simulink model "modelo_f_HIL"  (R2024b)
settings: Solver=ode15s  StartTime=0.0  StopTime=inf  FixedStep=T_s  RelTol=1e-3
InitFcn:
  | clc
  | clear
  | close all
  | clear all
  | clear mex
  | parametros
  | gain_CL
  | calculo_observador_carro
  | calculo_observador_izaje
values from neighbouring files (symbols this model uses):
  b_cx = 1e6    (= 1000000)    [parametros.m]
  b_cy = 1e7    (= 10000000)    [parametros.m]
  b_hb = 1e8    (= 100000000)    [parametros.m]
  b_hd = 8    [parametros.m]
  b_hm = 18    [parametros.m]
  b_t = 90    [parametros.m]
  b_tb = 5e6    (= 5000000)    [parametros.m]
  b_td = 1.8    [parametros.m]
  b_tm = 6    [parametros.m]
  b_tw = 3e3    (= 3000)    [parametros.m]
  b_wu = 150    [parametros.m]
  container_pillars = container_pillars(randperm(19))    [parametros.m]
  escenario = 1    [parametros.m]
  g = 9.80665    [parametros.m]
  H_c = 2.59    [parametros.m]
  H_truck = 1    [parametros.m]
  i_h = 22    [parametros.m]
  i_t = 30    [parametros.m]
  J_hd_hEb = 3800    [parametros.m]
  J_hm_hb = 30    [parametros.m]
  J_td = 1200    [parametros.m]
  J_tm_tb = 7    [parametros.m]
  K_cy = 1.8e9    (= 1800000000)    [parametros.m]
  K_tw = 4.8e5    (= 480000)    [parametros.m]
  k_wu = 2.36e8    (= 236000000)    [parametros.m]
  l_h0 = (Y_t0-y_l0)    (= 15)    [parametros.m]
  l_h_max = Y_t0-y_h_min    (= 65)    [parametros.m]
  l_h_maxE = l_h_max+0.5    (= 65.5)    [parametros.m]
  l_h_min = Y_t0-y_h_max    (= 5)    [parametros.m]
  l_h_minE = l_h_min-0.5    (= 4.5)    [parametros.m]
  M_cmax = 50000    [parametros.m]
  M_cmin = 2000    [parametros.m]
  M_s = 15000    [parametros.m]
  M_t = 30000    [parametros.m]
  r_hd = 0.75    [parametros.m]
  r_td = 0.50    (= 0.5)    [parametros.m]
  T_hbMax = 5e4    (= 50000)    [parametros.m]
  T_hEbMax = 1.1e6    (= 1100000)    [parametros.m]
  T_hmMax = 2e4    (= 20000)    [parametros.m]
  T_s = 0.001    [parametros.m]
  T_s0 = 0.001    [parametros.m]
  T_s1 = 0.020    (= 0.02)    [parametros.m]
  T_s2 = 0.020    (= 0.02)    [parametros.m]
  T_tbMax = 5e3    (= 5000)    [parametros.m]
  T_tmMax = 4e3    (= 4000)    [parametros.m]
  tau_tm = 1e-3    (= 0.001)    [parametros.m]
  theta_hm0 = -l_h0*i_h*2/r_hd    (= -880)    [parametros.m]
  theta_tm0 = (x_t0)*i_t/r_td    (= -1500)    [parametros.m]
  trucks0 = [0, 0, 0, 0, 0]    [parametros.m]
  v_h_max_load = 1.5    [parametros.m]
  v_h_max_noload = 3    [parametros.m]
  v_lx0 = 0    [parametros.m]
  v_ly0 = 0    [parametros.m]
  v_t0 = 0    [parametros.m]
  v_t_max = 4    [parametros.m]
  W_c = ctrb(A, B_c(:,1))    [CyO_carro.m]    (also in CyO_izaje.m; parametros.m = 2.44)
  w_hm0 = 0    [parametros.m]
  w_hm_rated = v_h_max_load*2*i_h/r_hd    (= 88)    [parametros.m]
  w_tm0 = (v_t0)*i_t/r_td    (= 0)    [parametros.m]
  x_c0_left = -35    [parametros.m]
  x_c0_right = 55    [parametros.m]
  x_containers_left_lim = 1.5    [parametros.m]
  x_containers_right_lim = 48.5    [parametros.m]
  x_l0 = x_t0    (= -25)    [parametros.m]
  x_lidar_offset = 3.0    (= 3)    [parametros.m]
  x_t0 = -25    [parametros.m]
  x_t_max = 50    [parametros.m]
  x_t_maxE = x_t_max+0.5    (= 50.5)    [parametros.m]
  x_t_min = -30    [parametros.m]
  x_t_minE = x_t_min-0.5    (= -30.5)    [parametros.m]
  y_h_min = -20    [parametros.m]
  y_l0 = 30    [parametros.m]
  Y_sb = 5.0    (= 5)    [parametros.m]
  Y_t0 = 45    [parametros.m]
libraries: opcualib x2, dspnetwork x2, dspsigops x1, simulink x1
(part 1 of 3)
settings Model: Creator=Usuario  LastModifiedBy=Usuario
settings RTWCC: GPUComputeCapability=3.5

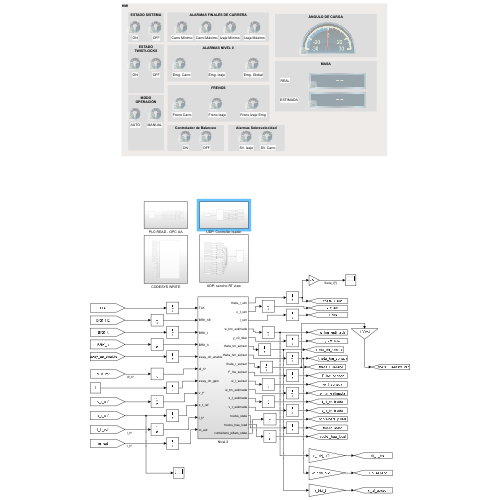
[thumbnail: Simulink's stored preview of the top-level diagram]
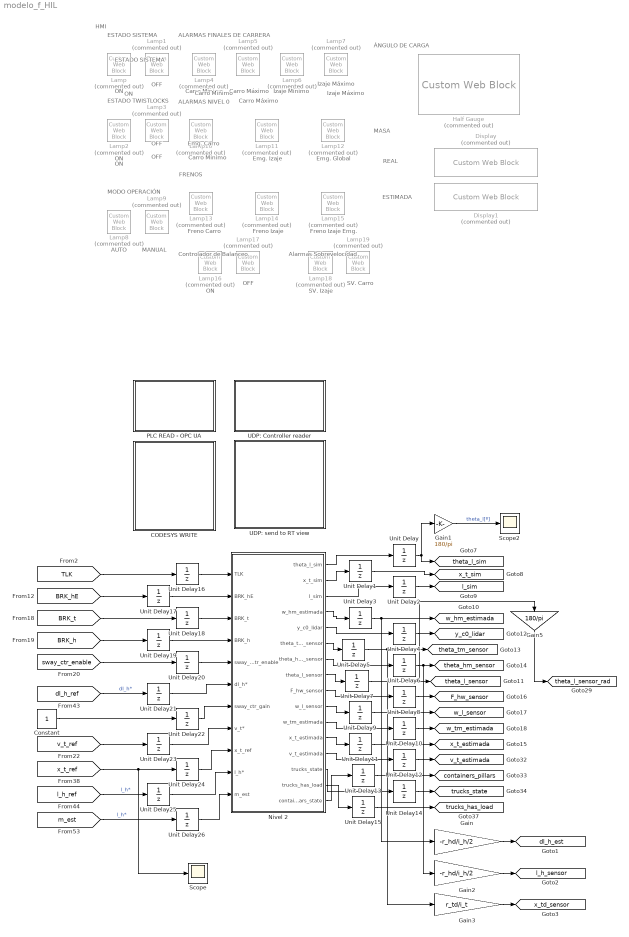
== system modelo_f_HIL ==
  note: ESTIMADA
  note: REAL
  note: OFF
  note: ON
  note: ESTADO SISTEMA
  note: HMI
  note: ON
  note: ESTADO SISTEMA
  note: ESTADO TWISTLOCKS
  note: OFF
  note: ON
  note: ON
  note: OFF
  note: Carro Mínimo
  note: ALARMAS FINALES DE CARRERA
  note: Carro Máximo
  note: Izaje Mínimo
  note: Izaje Máximo
  note: MANUAL
  note: AUTO
  note: MODO
      | OPERACIÓN
  note: Emg. Izaje
  note: ALARMAS NIVEL 0
  note: Carro Mínimo
  note: Izaje Máximo
  note: Carro Máximo
  note: Carro Mínimo
  note: Emg. Carro
  note: Emg. Global
  note: Freno Izaje Emg.
  note: Freno Carro
  note: FRENOS
  note: Freno Izaje
  note: OFF
  note: ON
  note: Controlador de Balanceo
  note: ÁNGULO DE CARGA
  note: MASA
  note: Alarmas Sobrevelocidad
  note: SV. Izaje
  note: SV. Carro
  CODESYS WRITE : Subsystem
  Constant : Constant
  Display : CustomWebBlock  Commented=on  LabelPosition=Hide  ShowInitialText=on  Configuration="{\"components\":[{\"name\":\"DisplayComponent\",\"settings\":{\"bold\":false,\"font\":\"DSEG7 Classic\",\"fontColor\":[255,255,200],\"fontSize\":\"14\",\"format\":\"short\",\"formatString\":\"%d\",\"italic\":false,\"position\":[0,0,1,1],\"underline\":false}},{\"name\":\"BackgroundImageComponent\",\"settings\":{\"image\":{\"size\":[300,80],\"src\":\"data:image\\/svg+xml;base64,PHN2ZyBpZD0iZnJhbWUiIHhtbG5zPSJodHRwOi8vd3d3LnczLm9yZy8yMDAwL3N2ZyIgeG1sbnM6eGxpbms9Imh0dHA6Ly93d3cudzMub3JnLzE5OTkveGxpbmsiIHZpZXdCb3g9IjAgMCAzODAgMTAxIj48ZGVmcz48c3R5bGU+LmNscy0xe2ZpbGw6IzAwMmI0Mjt9LmNscy0ye2ZpbGw6IzQyNzA4Mjt9LmNscy0ze2ZpbGw6dXJsKCNyYWRpYWwtZ3JhZGllbnQpO308L3N0eWxlPjxyYWRpYWxHcmFkaWVudCBpZD0icmFkaWFsLWdyYWRpZW50IiBjeD0iMTkwIiBjeT0iNTAuNSIgcj0iMjY5LjIxIiBncmFkaWVudFVuaXRzPSJ1c2VyU3BhY2VPblVzZSI+PHN0b3Agb2Zmc2V0PSIwLjAxIiBzdG9wLWNvbG9yPSIjM2U0ZjU4Ii8+PHN0b3Agb2Zmc2V0PSIwLjA2IiBzdG9wLWNvbG9yPSIjNDQ1NzYxIi8+PHN0b3Agb2Zmc2V0PSIwLjE1IiBzdG9wLWNvbG9yPSIjNTU2YTc2Ii8+PHN0b3Agb2Zmc2V0PSIwLjI1IiBzdG9wLWNvbG9yPSIjNmQ4ODk1Ii8+PHN0b3Agb2Zmc2V0PSIwLjM4IiBzdG9wLWNvbG9yPSIjOGZiMmMzIi8+PHN0b3Agb2Zmc2V0PSIwLjUyIiBzdG9wLWNvbG9yPSIjYjZlNGZhIi8+PHN0b3Agb2Zmc2V0PSIxIiBzdG9wLWNvbG9yPSIjMTU0NjU3Ii8+PC9yYWRpYWxHcmFkaWVudD48L2RlZnM+PGcgaWQ9IkxheWVyXzIiIGRhdGEtbmFtZT0iTGF5ZXIgMiI+PGcgaWQ9IkxheWVyXzEtMiIgZGF0YS1uYW1lPSJMYXllciAxLTIiPjxyZWN0IGlkPSJyZWN0MTAzNiIgY2xhc3M9ImNscy0xIiB4PSIxMSIgeT0iMTEiIHdpZHRoPSIzNTgiIGhlaWdodD0iNzkiLz48cGF0aCBpZD0icGF0aDEwMzgiIGNsYXNzPSJjbHMtMiIgZD0iTTgsOFY5M0gzNzJWOFpNMzY5LDkwSDExVjExSDM2OVoiLz48cGF0aCBpZD0icGF0aDEwNDAiIGNsYXNzPSJjbHMtMyIgZD0iTTAsMFYxMDFIMzgwVjBaTTM3Miw5M0g4VjhIMzcyWiIvPjwvZz48L2c+PC9zdmc+\",\"srcOrientation\":\"Right\"},\"position\":[0,0,1,1],\"scaleMode\":\"0\"}},{\"name\":\"ForegroundImageComponent\",\"settings\":{\"angle\":0,\"image\":{\"size\":[0,0],\"src\":\"default\"},\"isForeground\":1,\"position\":[0,0,1,1],\"scaleMode\":\"0\"}}],\"settings\":{\"BindingType\":\"signal\",\"aspectRatio\":1.032258064516129,\"backgroundColor\":[0,0,0,\"1\"],\"backgroundOffset\":0.14,\"backgroundOpacity\":1,\"fixedAspectRatio\":\"on\",\"showBackgroundColor\":false,\"value\":0,\"version\":\"R2023b\"},\"type\":\"Display\"}"
  Display1 : CustomWebBlock  Commented=on  LabelPosition=Hide  ShowInitialText=on  Configuration="{\"components\":[{\"name\":\"DisplayComponent\",\"settings\":{\"bold\":false,\"font\":\"DSEG7 Classic\",\"fontColor\":[255,255,200],\"fontSize\":\"14\",\"format\":\"short\",\"formatString\":\"%d\",\"italic\":false,\"position\":[0,0,1,1],\"underline\":false}},{\"name\":\"BackgroundImageComponent\",\"settings\":{\"image\":{\"size\":[300,80],\"src\":\"data:image\\/svg+xml;base64,PHN2ZyBpZD0iZnJhbWUiIHhtbG5zPSJodHRwOi8vd3d3LnczLm9yZy8yMDAwL3N2ZyIgeG1sbnM6eGxpbms9Imh0dHA6Ly93d3cudzMub3JnLzE5OTkveGxpbmsiIHZpZXdCb3g9IjAgMCAzODAgMTAxIj48ZGVmcz48c3R5bGU+LmNscy0xe2ZpbGw6IzAwMmI0Mjt9LmNscy0ye2ZpbGw6IzQyNzA4Mjt9LmNscy0ze2ZpbGw6dXJsKCNyYWRpYWwtZ3JhZGllbnQpO308L3N0eWxlPjxyYWRpYWxHcmFkaWVudCBpZD0icmFkaWFsLWdyYWRpZW50IiBjeD0iMTkwIiBjeT0iNTAuNSIgcj0iMjY5LjIxIiBncmFkaWVudFVuaXRzPSJ1c2VyU3BhY2VPblVzZSI+PHN0b3Agb2Zmc2V0PSIwLjAxIiBzdG9wLWNvbG9yPSIjM2U0ZjU4Ii8+PHN0b3Agb2Zmc2V0PSIwLjA2IiBzdG9wLWNvbG9yPSIjNDQ1NzYxIi8+PHN0b3Agb2Zmc2V0PSIwLjE1IiBzdG9wLWNvbG9yPSIjNTU2YTc2Ii8+PHN0b3Agb2Zmc2V0PSIwLjI1IiBzdG9wLWNvbG9yPSIjNmQ4ODk1Ii8+PHN0b3Agb2Zmc2V0PSIwLjM4IiBzdG9wLWNvbG9yPSIjOGZiMmMzIi8+PHN0b3Agb2Zmc2V0PSIwLjUyIiBzdG9wLWNvbG9yPSIjYjZlNGZhIi8+PHN0b3Agb2Zmc2V0PSIxIiBzdG9wLWNvbG9yPSIjMTU0NjU3Ii8+PC9yYWRpYWxHcmFkaWVudD48L2RlZnM+PGcgaWQ9IkxheWVyXzIiIGRhdGEtbmFtZT0iTGF5ZXIgMiI+PGcgaWQ9IkxheWVyXzEtMiIgZGF0YS1uYW1lPSJMYXllciAxLTIiPjxyZWN0IGlkPSJyZWN0MTAzNiIgY2xhc3M9ImNscy0xIiB4PSIxMSIgeT0iMTEiIHdpZHRoPSIzNTgiIGhlaWdodD0iNzkiLz48cGF0aCBpZD0icGF0aDEwMzgiIGNsYXNzPSJjbHMtMiIgZD0iTTgsOFY5M0gzNzJWOFpNMzY5LDkwSDExVjExSDM2OVoiLz48cGF0aCBpZD0icGF0aDEwNDAiIGNsYXNzPSJjbHMtMyIgZD0iTTAsMFYxMDFIMzgwVjBaTTM3Miw5M0g4VjhIMzcyWiIvPjwvZz48L2c+PC9zdmc+\",\"srcOrientation\":\"Right\"},\"position\":[0,0,1,1],\"scaleMode\":\"0\"}},{\"name\":\"ForegroundImageComponent\",\"settings\":{\"angle\":0,\"image\":{\"size\":[0,0],\"src\":\"default\"},\"isForeground\":1,\"position\":[0,0,1,1],\"scaleMode\":\"0\"}}],\"settings\":{\"BindingType\":\"signal\",\"aspectRatio\":1.032258064516129,\"backgroundColor\":[0,0,0,\"1\"],\"backgroundOffset\":0.14,\"backgroundOpacity\":1,\"fixedAspectRatio\":\"on\",\"showBackgroundColor\":false,\"value\":0,\"version\":\"R2023b\"},\"type\":\"Display\"}"
  Gain : Gain  Gain=-r_hd/i_h/2
  Gain1 : Gain  Gain=180/pi
  Gain2 : Gain  Gain=-r_hd/i_h/2
  Gain3 : Gain  Gain=r_td/i_t
  Gain5 : Gain  Gain=180/pi
  Half Gauge : CustomWebBlock  Commented=on  LabelPosition=Hide  ShowInitialText=on  Configuration="{\"components\":[{\"name\":\"CircularScaleComponent\",\"settings\":{\"bounds\":{\"max\":30,\"min\":-30,\"tickInterval\":\"auto\"},\"direction\":\"cw\",\"flipLimits\":0,\"innerRadius\":0.75,\"internalTickHeightScaleFactor\":1,\"labelColor\":[255,255,200],\"labelFont\":{\"font\":\"Arial\",\"fontSize\":12},\"labelRadius\":0.528,\"labelTransparency\":1,\"minorTickHeightScaleFactor\":0.2,\"needleImage\":{\"size\":[200,50],\"src\":\"data:image\\/svg+xml;base64,PD94bWwgdmVyc2lvbj0iMS4wIiBlbmNvZGluZz0idXRmLTgiPz4KPCEtLSBHZW5lcmF0b3I6IEFkb2JlIElsbHVzdHJhdG9yIDI0LjEuMiwgU1ZHIEV4cG9ydCBQbHVnLUluIC4gU1ZHIFZlcnNpb246IDYuMDAgQnVpbGQgMCkgIC0tPgo8c3ZnIHZlcnNpb249IjEuMSIgaWQ9IkxheWVyXzEiIHhtbG5zPSJodHRwOi8vd3d3LnczLm9yZy8yMDAwL3N2ZyIgeG1sbnM6eGxpbms9Imh0dHA6Ly93d3cudzMub3JnLzE5OTkveGxpbmsiIHg9IjBweCIgeT0iMHB4IgoJIHZpZXdCb3g9IjAgMCAyMDAgNTAiIHN0eWxlPSJlbmFibGUtYmFja2dyb3VuZDpuZXcgMCAwIDIwMCA1MDsiIHhtbDpzcGFjZT0icHJlc2VydmUiPgo8c3R5bGUgdHlwZT0idGV4dC9jc3MiPgoJLnN0MHtmaWxsOiNFQzIxMjc7fQo8L3N0eWxlPgo8cGF0aCBjbGFzcz0ic3QwIiBkPSJNMTYyLjgsMTMuN0MxNjksNC40LDE4MS43LDEuOSwxOTEsOC4xczExLjgsMTguOSw1LjYsMjguMnMtMTguOSwxMS44LTI4LjIsNS42bDAsMAoJQzE1OS4xLDM1LjYsMTU2LjYsMjMsMTYyLjgsMTMuN0wxNjIuOCwxMy43eiBNMTY1LjgsMTUuOGMtNS4xLDcuNi0zLjEsMTcuOSw0LjYsMjNjNy42LDUuMSwxNy45LDMuMSwyMy00LjYKCWM1LjEtNy42LDMuMS0xNy45LTQuNi0yM2wwLDBDMTgxLjIsNi4yLDE3MC45LDguMiwxNjUuOCwxNS44eiIvPgo8cGF0aCBjbGFzcz0ic3QwIiBkPSJNMC40LDI1Ljl2LTMuM2wxNTktMi41Yy0wLjcsMi42LTAuNyw1LjIsMCw3LjhMMC40LDI1Ljl6Ii8+CjxjaXJjbGUgY2xhc3M9InN0MCIgY3g9IjE3OS42IiBjeT0iMjQiIHI9IjAuNyIvPgo8L3N2Zz4K\"},\"needleOffset\":[0.18464878250906522,0],\"needleOrientation\":-45,\"needleRotation\":180,\"needleSize\":{\"height\":0.11741692305346914,\"width\":0.46108337545091255},\"outerRadius\":0.9,\"position\":[0.05,0.05,0.9,1.6],\"referencePoint\":\"auto\",\"scaleAngle\":180,\"scaleAngleOffset\":180,\"scaleColors\":[],\"scaleColorsSize\":0.2,\"scaleDirection\":\"CW\",\"scalePosition\":[0,0,1,1],\"showLabels\":1,\"showMinorTicks\":1,\"showSpanLine\":1,\"showTicks\":1,\"tickColor\":[252,252,197],\"tickTransparency\":1,\"valueBarColor\":[0,114,189],\"valueBarPosition\":[0,0,1,1],\"valueBarSize\":0.2,\"valueBarTransparency\":1}},{\"name\":\"BackgroundImageComponent\",\"settings\":{\"image\":{\"size\":[252,150],\"src\":\"data:image\\/svg+xml;base64,PD94bWwgdmVyc2lvbj0iMS4wIiBlbmNvZGluZz0idXRmLTgiPz4KPCEtLSBHZW5lcmF0b3I6IEFkb2JlIElsbHVzdHJhdG9yIDI2LjEuMCwgU1ZHIEV4cG9ydCBQbHVnLUluIC4gU1ZHIFZlcnNpb246IDYuMDAgQnVpbGQgMCkgIC0tPgo8c3ZnIHZlcnNpb249IjEuMSIKCSBpZD0iTGF5ZXJfMl8xXyIgeG1sbnM6Y2M9Imh0dHA6Ly9jcmVhdGl2ZWNvbW1vbnMub3JnL25zIyIgeG1sbnM6ZGM9Imh0dHA6Ly9wdXJsLm9yZy9kYy9lbGVtZW50cy8xLjEvIiB4bWxuczppbmtzY2FwZT0iaHR0cDovL3d3dy5pbmtzY2FwZS5vcmcvbmFt ...(+5492 chars)\",\"srcOrientation\":\"Right\"},\"position\":[0,0,1,1],\"scaleMode\":\"0\"}},{\"name\":\"ForegroundImageComponent\",\"settings\":{\"image\":{\"size\":[0,0],\"src\":\"default\",\"srcOrientation\":[]},\"isForeground\":1,\"position\":[0,0,1,1],\"scaleMode\":\"0\"}}],\"settings\":{\"BindingType\":\"signal\",\"aspectRatio\":1.032258064516129,\"backgroundColor\":[0,0,0,\"1\"],\"backgroundOffset\":1,\"backgroundOpacity\":1,\"direction\":\"cw\",\"fixedAspectRatio\":\"on\",\"flipLimits\":0,\"orientation\":\"horizontal\",\"showBackgroundColor\":false,\"value\":0,\"variant\":\"half\",\"version\":\"R2023a\"},\"type\":\"CircularGauge\"}"
  Lamp{,2,4..8,10..12,16,18..19} (13 alike) : CustomWebBlock  Commented=on  LabelPosition=Hide  ShowInitialText=on  Configuration="{\"components\":[{\"name\":\"BackgroundImageComponent\",\"settings\":{\"image\":{\"size\":[150,150],\"src\":\"data:image\\/svg+xml;base64,PHN2ZyB4bWxucz0iaHR0cDovL3d3dy53My5vcmcvMjAwMC9zdmciIHhtbG5zOnhsaW5rPSJodHRwOi8vd3d3LnczLm9yZy8xOTk5L3hsaW5rIiB2aWV3Qm94PSIwIDAgNTAwIDUwMCI+PGRlZnM+PHN0eWxlPi5he2ZpbGw6dXJsKCNhKTt9LmJ7ZmlsbDp1cmwoI2IpO30uY3tmaWxsOnVybCgjYyk7fTwvc3R5bGU+PHJhZGlhbEdyYWRpZW50IGlkPSJhIiBjeD0iMjgzLjg0IiBjeT0iLTQ2Ni4zNyIgcj0iMzc1Ljc1IiBncmFkaWVudFRyYW5zZm9ybT0ibWF0cml4KDEuMzksIDAsIDAsIC0xLjM5LCAtMTUzLjU2LCAtNjQ0LjA4KSIg ...(+2088 chars)\",\"srcOrientation\":\"Right\"},\"position\":[0,0,1,1],\"scaleMode\":\"0\"}},{\"name\":\"LampStateComponent\",\"settings\":{\"position\":[0,0,1,1],\"states\":[{\"icon\":{\"customSrc\":\"data:image\\/svg+xml;base64,PHN2ZyBpZD0iTGF5ZXJfMSIgZGF0YS1uYW1lPSJMYXllciAxIiB4bWxucz0iaHR0cDovL3d3dy53My5vcmcvMjAwMC9zdmciIHZpZXdCb3g9IjAgMCA0MTEgNDU4Ij48ZGVmcz48c3R5bGU+LmNscy0xe2ZpbGw6I2ZkZjhjMTt9LmNscy0ye2ZpbGw6I2ZlZTEwMDt9LmNscy0ze2ZpbGw6IzIzMWYyMDt9LmNscy00e2ZpbGw6I2EwOWY5Zjt9LmNscy00LC5jbHMtNSwuY2xzLTZ7c3Ryb2tlOiMyMzFmMjA7c3Ryb2tlLW1pdGVybGltaXQ6MTA7fS5jbHMtNXtmaWxsOiNmZmY7fS5jbHMtNntmaWxsOm5vbmU7fTwvc3R5bGU+PC9kZWZz ...(+5168 chars)\",\"id\":-1,\"srcOrientation\":\"Right\",\"type\":\"custom\"},\"iconScale\":0.8,\"metadata\":{},\"overlayType\":\"intersect\",\"shape\":{\"color\":[0.8,0.8,0.8],\"opacity\":1,\"position\":[0.1,0.1,0.8,0.8],\"type\":\"ellipse\"},\"value\":[]},{\"icon\":{\"customSrc\":\"data:image\\/svg+xml;base64,PHN2ZyBpZD0iTGF5ZXJfMSIgZGF0YS1uYW1lPSJMYXllciAxIiB4bWxucz0iaHR0cDovL3d3dy53My5vcmcvMjAwMC9zdmciIHZpZXdCb3g9IjAgMCA0MTEgNDU4Ij48ZGVmcz48c3R5bGU+LmNscy0xe2ZpbGw6I2ZkZjhjMTt9LmNscy0ye2ZpbGw6I2ZlZTEwMDt9LmNscy0ze2ZpbGw6IzIzMWYyMDt9LmNscy00e2ZpbGw6I2EwOWY5Zjt9LmNscy00LC5jbHMtNSwuY2xzLTZ7c3Ryb2tlOiMyMzFmMjA7c3Ryb2tlLW1pdGVybGltaXQ6MTA7fS5jbHMtNXtmaWxsOiNmZmY7fS5jbHMtNntmaWxsOm5vbmU7fTwvc3R5bGU+PC9kZWZz ...(+5168 chars)\",\"id\":-1,\"srcOrientation\":\"Right\",\"type\":\"custom\"},\"iconScale\":0.8,\"metadata\":{\"useDefaults\":{\"customIcon\":true,\"icon\":true,\"overlayType\":true,\"shape\":true,\"sizeAndPosition\":true}},\"overlayType\":\"intersect\",\"shape\":{\"color\":[0.8,0.8,0.8],\"opacity\":1,\"position\":[0.1,0.1,0.8,0.8],\"type\":\"ellipse\"},\"value\":\"0\"},{\"icon\":{\"customSrc\":\"data:image\\/svg+xml;base64,PHN2ZyBpZD0iTGF5ZXJfMSIgZGF0YS1uYW1lPSJMYXllciAxIiB4bWxucz0iaHR0cDovL3d3dy53My5vcmcvMjAwMC9zdmciIHZpZXdCb3g9IjAgMCA0MTEgNDU4Ij48ZGVmcz48c3R5bGU+LmNscy0xe2ZpbGw6I2ZkZjhjMTt9LmNscy0ye2ZpbGw6I2ZlZTEwMDt9LmNscy0ze2ZpbGw6IzIzMWYyMDt9LmNscy00e2ZpbGw6I2EwOWY5Zjt9LmNscy00LC5jbHMtNSwuY2xzLTZ7c3Ryb2tlOiMyMzFmMjA7c3Ryb2tlLW1pdGVybGltaXQ6MTA7fS5jbHMtNXtmaWxsOiNmZmY7fS5jbHMtNntmaWxsOm5vbmU7fTwvc3R5bGU+PC9kZWZz ...(+5168 chars)\",\"id\":-1,\"srcOrientation\":\"Right\",\"type\":\"custom\"},\"iconScale\":0.8,\"metadata\":{\"useDefaults\":{\"customIcon\":true,\"icon\":true,\"overlayType\":true,\"shape\":true,\"sizeAndPosition\":true}},\"overlayType\":\"intersect\",\"shape\":{\"color\":[0,1,0],\"opacity\":1,\"position\":[0.1,0.1,0.8,0.8],\"type\":\"ellipse\"},\"value\":\"1\"}],\"valueType\":\"discrete\"}},{\"name\":\"ForegroundImageComponent\",\"settings\":{\"image\":{\"size\":[150,150],\"src\":\"data:image\\/svg+xml;base64,PHN2ZyB4bWxucz0iaHR0cDovL3d3dy53My5vcmcvMjAwMC9zdmciIHhtbG5zOnhsaW5rPSJodHRwOi8vd3d3LnczLm9yZy8xOTk5L3hsaW5rIiB2aWV3Qm94PSIwIDAgNTAwIDUwMCI+PGRlZnM+PHN0eWxlPi5he2ZpbGw6dXJsKCNhKTt9PC9zdHlsZT48bGluZWFyR3JhZGllbnQgaWQ9ImEiIHgxPSIxNzMuMDUiIHkxPSItNjI3Ljc4IiB4Mj0iMTczLjA1IiB5Mj0iLTUyMi40MyIgZ3JhZGllbnRUcmFuc2Zvcm09Im1hdHJpeCgxLjI5LCAwLCAwLCAtMS4zMywgMjcuMTMsIC02MjguMzEpIiBncmFkaWVudFVuaXRzPSJ1c2VyU3BhY2VPblVzZSI+PHN0b3Agb2Zmc2V0PSIwIiBzdG9wLWNvbG9yPSIjZmZmIiBzdG9wLW9wYWNpdHk9IjAuMjUiLz48c3RvcCBvZmZzZXQ9IjEiIHN0b3AtY29sb3I9IiNmZmYiIHN0b3Atb3BhY2l0eT0iMCIvPjwvbGluZWFyR3JhZGllbnQ+PC9kZWZzPjxwYXRoIGNsYXNzPSJhIiBkPSJNNDI5LjMsMTkwLjY2QzQwMi40NSwxMTQuNTEsMzMyLjY3LDYwLjE3LDI1MC44NSw2MC4xN2MtODMuNDMsMC0xNTQuMjgsNTYuNDItMTc5Ljk1LDEzNSwxNS4zNCwzOSw4OC4xMSw3LDE3Ny4wNyw3QzM0MCwyMDIuMDgsNDE3LjI2LDIzNi40Niw0MjkuMywxOTAuNjZaIi8+PC9zdmc+\",\"srcOrientation\":\"Right\"},\"isForeground\":1,\"position\":[0,0,1,1],\"scaleMode\":\"0\"}}],\"settings\":{\"BindingType\":\"signal\",\"aspectRatio\":1.032258064516129,\"backgroundColor\":[0,0,0],\"backgroundOffset\":0.14,\"backgroundOpacity\":1,\"blockOrientation\":\"Right\",\"fixedAspectRatio\":\"on\",\"showBackgroundColor\":false,\"value\":0,\"version\":\"R2023a\"},\"type\":\"Lamp\"}"  StateValueType=Discrete  Icon=Custom
  Lamp{1,3,9,13..15,17} (7 alike) : CustomWebBlock  Commented=on  LabelPosition=Hide  ShowInitialText=on  Configuration="{\"components\":[{\"name\":\"BackgroundImageComponent\",\"settings\":{\"image\":{\"size\":[150,150],\"src\":\"data:image\\/svg+xml;base64,PHN2ZyB4bWxucz0iaHR0cDovL3d3dy53My5vcmcvMjAwMC9zdmciIHhtbG5zOnhsaW5rPSJodHRwOi8vd3d3LnczLm9yZy8xOTk5L3hsaW5rIiB2aWV3Qm94PSIwIDAgNTAwIDUwMCI+PGRlZnM+PHN0eWxlPi5he2ZpbGw6dXJsKCNhKTt9LmJ7ZmlsbDp1cmwoI2IpO30uY3tmaWxsOnVybCgjYyk7fTwvc3R5bGU+PHJhZGlhbEdyYWRpZW50IGlkPSJhIiBjeD0iMjgzLjg0IiBjeT0iLTQ2Ni4zNyIgcj0iMzc1Ljc1IiBncmFkaWVudFRyYW5zZm9ybT0ibWF0cml4KDEuMzksIDAsIDAsIC0xLjM5LCAtMTUzLjU2LCAtNjQ0LjA4KSIg ...(+2088 chars)\",\"srcOrientation\":\"Right\"},\"position\":[0,0,1,1],\"scaleMode\":\"0\"}},{\"name\":\"LampStateComponent\",\"settings\":{\"position\":[0,0,1,1],\"states\":[{\"icon\":{\"customSrc\":\"data:image\\/svg+xml;base64,PHN2ZyBpZD0iTGF5ZXJfMSIgZGF0YS1uYW1lPSJMYXllciAxIiB4bWxucz0iaHR0cDovL3d3dy53My5vcmcvMjAwMC9zdmciIHZpZXdCb3g9IjAgMCA0MTEgNDU4Ij48ZGVmcz48c3R5bGU+LmNscy0xe2ZpbGw6I2ZkZjhjMTt9LmNscy0ye2ZpbGw6I2ZlZTEwMDt9LmNscy0ze2ZpbGw6IzIzMWYyMDt9LmNscy00e2ZpbGw6I2EwOWY5Zjt9LmNscy00LC5jbHMtNSwuY2xzLTZ7c3Ryb2tlOiMyMzFmMjA7c3Ryb2tlLW1pdGVybGltaXQ6MTA7fS5jbHMtNXtmaWxsOiNmZmY7fS5jbHMtNntmaWxsOm5vbmU7fTwvc3R5bGU+PC9kZWZz ...(+5168 chars)\",\"id\":-1,\"srcOrientation\":\"Right\",\"type\":\"custom\"},\"iconScale\":0.8,\"metadata\":{},\"overlayType\":\"intersect\",\"shape\":{\"color\":[0.8,0.8,0.8],\"opacity\":1,\"position\":[0.1,0.1,0.8,0.8],\"type\":\"ellipse\"},\"value\":[]},{\"icon\":{\"customSrc\":\"data:image\\/svg+xml;base64,PHN2ZyBpZD0iTGF5ZXJfMSIgZGF0YS1uYW1lPSJMYXllciAxIiB4bWxucz0iaHR0cDovL3d3dy53My5vcmcvMjAwMC9zdmciIHZpZXdCb3g9IjAgMCA0MTEgNDU4Ij48ZGVmcz48c3R5bGU+LmNscy0xe2ZpbGw6I2ZkZjhjMTt9LmNscy0ye2ZpbGw6I2ZlZTEwMDt9LmNscy0ze2ZpbGw6IzIzMWYyMDt9LmNscy00e2ZpbGw6I2EwOWY5Zjt9LmNscy00LC5jbHMtNSwuY2xzLTZ7c3Ryb2tlOiMyMzFmMjA7c3Ryb2tlLW1pdGVybGltaXQ6MTA7fS5jbHMtNXtmaWxsOiNmZmY7fS5jbHMtNntmaWxsOm5vbmU7fTwvc3R5bGU+PC9kZWZz ...(+5168 chars)\",\"id\":-1,\"srcOrientation\":\"Right\",\"type\":\"custom\"},\"iconScale\":0.8,\"metadata\":{\"useDefaults\":{\"customIcon\":true,\"icon\":true,\"overlayType\":true,\"shape\":true,\"sizeAndPosition\":true}},\"overlayType\":\"intersect\",\"shape\":{\"color\":[0,1,0],\"opacity\":1,\"position\":[0.1,0.1,0.8,0.8],\"type\":\"ellipse\"},\"value\":\"0\"},{\"icon\":{\"customSrc\":\"data:image\\/svg+xml;base64,PHN2ZyBpZD0iTGF5ZXJfMSIgZGF0YS1uYW1lPSJMYXllciAxIiB4bWxucz0iaHR0cDovL3d3dy53My5vcmcvMjAwMC9zdmciIHZpZXdCb3g9IjAgMCA0MTEgNDU4Ij48ZGVmcz48c3R5bGU+LmNscy0xe2ZpbGw6I2ZkZjhjMTt9LmNscy0ye2ZpbGw6I2ZlZTEwMDt9LmNscy0ze2ZpbGw6IzIzMWYyMDt9LmNscy00e2ZpbGw6I2EwOWY5Zjt9LmNscy00LC5jbHMtNSwuY2xzLTZ7c3Ryb2tlOiMyMzFmMjA7c3Ryb2tlLW1pdGVybGltaXQ6MTA7fS5jbHMtNXtmaWxsOiNmZmY7fS5jbHMtNntmaWxsOm5vbmU7fTwvc3R5bGU+PC9kZWZz ...(+5168 chars)\",\"id\":-1,\"srcOrientation\":\"Right\",\"type\":\"custom\"},\"iconScale\":0.8,\"metadata\":{\"useDefaults\":{\"customIcon\":true,\"icon\":true,\"overlayType\":true,\"shape\":true,\"sizeAndPosition\":true}},\"overlayType\":\"intersect\",\"shape\":{\"color\":[0.8,0.8,0.8],\"opacity\":1,\"position\":[0.1,0.1,0.8,0.8],\"type\":\"ellipse\"},\"value\":\"1\"}],\"valueType\":\"discrete\"}},{\"name\":\"ForegroundImageComponent\",\"settings\":{\"image\":{\"size\":[150,150],\"src\":\"data:image\\/svg+xml;base64,PHN2ZyB4bWxucz0iaHR0cDovL3d3dy53My5vcmcvMjAwMC9zdmciIHhtbG5zOnhsaW5rPSJodHRwOi8vd3d3LnczLm9yZy8xOTk5L3hsaW5rIiB2aWV3Qm94PSIwIDAgNTAwIDUwMCI+PGRlZnM+PHN0eWxlPi5he2ZpbGw6dXJsKCNhKTt9PC9zdHlsZT48bGluZWFyR3JhZGllbnQgaWQ9ImEiIHgxPSIxNzMuMDUiIHkxPSItNjI3Ljc4IiB4Mj0iMTczLjA1IiB5Mj0iLTUyMi40MyIgZ3JhZGllbnRUcmFuc2Zvcm09Im1hdHJpeCgxLjI5LCAwLCAwLCAtMS4zMywgMjcuMTMsIC02MjguMzEpIiBncmFkaWVudFVuaXRzPSJ1c2VyU3BhY2VPblVzZSI+PHN0b3Agb2Zmc2V0PSIwIiBzdG9wLWNvbG9yPSIjZmZmIiBzdG9wLW9wYWNpdHk9IjAuMjUiLz48c3RvcCBvZmZzZXQ9IjEiIHN0b3AtY29sb3I9IiNmZmYiIHN0b3Atb3BhY2l0eT0iMCIvPjwvbGluZWFyR3JhZGllbnQ+PC9kZWZzPjxwYXRoIGNsYXNzPSJhIiBkPSJNNDI5LjMsMTkwLjY2QzQwMi40NSwxMTQuNTEsMzMyLjY3LDYwLjE3LDI1MC44NSw2MC4xN2MtODMuNDMsMC0xNTQuMjgsNTYuNDItMTc5Ljk1LDEzNSwxNS4zNCwzOSw4OC4xMSw3LDE3Ny4wNyw3QzM0MCwyMDIuMDgsNDE3LjI2LDIzNi40Niw0MjkuMywxOTAuNjZaIi8+PC9zdmc+\",\"srcOrientation\":\"Right\"},\"isForeground\":1,\"position\":[0,0,1,1],\"scaleMode\":\"0\"}}],\"settings\":{\"BindingType\":\"signal\",\"aspectRatio\":1.032258064516129,\"backgroundColor\":[0,0,0],\"backgroundOffset\":0.14,\"backgroundOpacity\":1,\"blockOrientation\":\"Right\",\"fixedAspectRatio\":\"on\",\"showBackgroundColor\":false,\"value\":0,\"version\":\"R2023a\"},\"type\":\"Lamp\"}"  StateValueType=Discrete  Icon=Custom
  Nivel 2 : Subsystem
  PLC READ - OPC UA : Subsystem
  Scope : Scope
  Scope2 : Scope
  UDP: Controller reader : Subsystem
  UDP: send to RT view : Subsystem
  Unit Delay{,3..4,7..10,12} (8 alike) : UnitDelay  SampleTime=T_s2  HasFrameUpgradeWarning=on
  Unit Delay1 : UnitDelay  InitialCondition=x_t0  SampleTime=T_s2  HasFrameUpgradeWarning=on
  Unit Delay11 : UnitDelay  InitialCondition=theta_tm0*r_td/i_t  SampleTime=T_s2  HasFrameUpgradeWarning=on
  Unit Delay13 : UnitDelay  InitialCondition=container_pillars  SampleTime=T_s2  HasFrameUpgradeWarning=on
  Unit Delay14 : UnitDelay  InitialCondition=trucks0  SampleTime=T_s2  HasFrameUpgradeWarning=on
  Unit Delay15 : UnitDelay  InitialCondition=trucks0  SampleTime=T_s2  HasFrameUpgradeWarning=on
  Unit Delay{16,21..23} (4 alike) : UnitDelay  SampleTime=T_s1  HasFrameUpgradeWarning=on
  Unit Delay17 : UnitDelay  InitialCondition=false  SampleTime=T_s1  HasFrameUpgradeWarning=on
  Unit Delay18 : UnitDelay  InitialCondition=false  SampleTime=T_s1  HasFrameUpgradeWarning=on
  Unit Delay19 : UnitDelay  InitialCondition=false  SampleTime=T_s1  HasFrameUpgradeWarning=on
  Unit Delay2 : UnitDelay  InitialCondition=l_h0  SampleTime=T_s2  HasFrameUpgradeWarning=on
  Unit Delay20 : UnitDelay  InitialCondition=true  SampleTime=T_s1  HasFrameUpgradeWarning=on
  Unit Delay24 : UnitDelay  InitialCondition=theta_tm0*r_td/i_t  SampleTime=T_s1  HasFrameUpgradeWarning=on
  Unit Delay25 : UnitDelay  InitialCondition=-theta_hm0*r_hd/i_h/2  SampleTime=T_s1  HasFrameUpgradeWarning=on
  Unit Delay26 : UnitDelay  InitialCondition=M_s  SampleTime=T_s1  HasFrameUpgradeWarning=on
  Unit Delay5 : UnitDelay  InitialCondition=theta_tm0  SampleTime=T_s2  StateName=theta_tm0  HasFrameUpgradeWarning=on
  Unit Delay6 : UnitDelay  InitialCondition=theta_hm0  SampleTime=T_s2  HasFrameUpgradeWarning=on
  tag scope: F_hw_sensor=global, containers_pillars=global, dl_h_est=global, l_h_sensor=global, l_sim=global, theta_hm_sensor=global, theta_l_sensor=global, theta_l_sensor_rad=global, theta_l_sim=global, theta_tm_sensor=global, trucks_has_load=global, trucks_state=global, v_t_estimada=global, w_hm_estimada=global, w_l_sensor=global, w_tm_estimada=global, x_t_estimada=global, x_t_sim=global, x_td_sensor=global, y_c0_lidar=global
  wires:
  Nivel 2/1(theta_l_sim) -> Unit Delay/1
  Nivel 2/12(x_t_estimada) -> Unit Delay11/1
  Nivel 2/11(w_tm_estimada) -> Unit Delay10/1
  Nivel 2/10(w_l_sensor) -> Unit Delay9/1
  Nivel 2/9(F_hw_sensor) -> Unit Delay8/1
  Nivel 2/7(theta_hm_sensor) -> Unit Delay6/1
  Nivel 2/8(theta_l_sensor) -> Unit Delay7/1
  Nivel 2/6(theta_tm_sensor) -> Unit Delay5/1
  Nivel 2/5(y_c0_lidar) -> Unit Delay4/1
  Nivel 2/4(w_hm_estimada) -> Unit Delay3/1
  Nivel 2/3(l_sim) -> Unit Delay2/1
  Nivel 2/2(x_t_sim) -> Unit Delay1/1
  [TLK] -> Unit Delay16/1
  [BRK_hE] -> Unit Delay17/1
  Unit Delay/1 -> [theta_l_sim], Gain1/1
  Unit Delay1/1 -> [x_t_sim]
  Unit Delay2/1 -> [l_sim]
  Unit Delay3/1 -> Gain/1, [w_hm_estimada]
  Unit Delay4/1 -> [y_c0_lidar]
  Unit Delay7/1 -> Gain5/1, [theta_l_sensor]
  Unit Delay6/1 -> Gain2/1, [theta_hm_sensor]
  Unit Delay5/1 -> Gain3/1, [theta_tm_sensor]
  Unit Delay10/1 -> [w_tm_estimada]
  Unit Delay11/1 -> [x_t_estimada]
  Unit Delay8/1 -> [F_hw_sensor]
  Unit Delay9/1 -> [w_l_sensor]
  [BRK_t] -> Unit Delay18/1
  [BRK_h] -> Unit Delay19/1
  [sway_ctr_enable] -> Unit Delay20/1
  [v_t_ref] -> Unit Delay23/1
  Nivel 2/13(v_t_estimada) -> Unit Delay12/1
  Unit Delay12/1 -> [v_t_estimada]
  [dl_h_ref] -> Unit Delay21/1  "dl_h*"
  Nivel 2/14(trucks_state) -> Unit Delay14/1
  Unit Delay13/1 -> [containers_pillars]
  Unit Delay14/1 -> [trucks_state]
  Nivel 2/15(trucks_has_load) -> Unit Delay15/1
  Unit Delay15/1 -> [trucks_has_load]
  Gain1/1 -> Scope2/1  "theta_l[º]"
  Constant/1 -> Unit Delay22/1
  [x_t_ref] -> Scope/1, Unit Delay24/1
  [l_h_ref] -> Unit Delay25/1  "l_h*"
  Nivel 2/16(containers_pillars_state) -> Unit Delay13/1
  Gain5/1 -> [theta_l_sensor_rad]
  [m_est] -> Unit Delay26/1  "l_h*"
  Gain/1 -> [dl_h_est]
  Gain2/1 -> [l_h_sensor]
  Gain3/1 -> [x_td_sensor]
  Unit Delay16/1 -> Nivel 2/1(TLK)
  Unit Delay17/1 -> Nivel 2/2(BRK_hE)
  Unit Delay18/1 -> Nivel 2/3(BRK_t)
  Unit Delay20/1 -> Nivel 2/5(sway_ctr_enable)
  Unit Delay19/1 -> Nivel 2/4(BRK_h)
  Unit Delay22/1 -> Nivel 2/7(sway_ctr_gain)
  Unit Delay21/1 -> Nivel 2/6(dl_h*)
  Unit Delay23/1 -> Nivel 2/8(v_t*)
  Unit Delay24/1 -> Nivel 2/9(x_t_ref)
  Unit Delay26/1 -> Nivel 2/11(m_est)
  Unit Delay25/1 -> Nivel 2/10(l_h*)
